simulink model "quadrotor"  (R2019a)
settings: Solver=ode4  StartTime=0.0  StopTime=inf  FixedStep=simparam_delta_t  RelTol=1e-3
model workspace (MAT data in the model file):
  simparam_I = Simulink.Parameter
  simparam_I.Value = [1  0  0; 0  1  0; 0  0  1]
  simparam_I.DataType = 'auto'
  simparam_I.Dimensions = [3 3]
  simparam_delta_t = Simulink.Parameter
  simparam_delta_t.Value = 0.01
  simparam_delta_t.DataType = 'auto'
  simparam_delta_t.Dimensions = [1 1]
  simparam_g = Simulink.Parameter
  simparam_g.Value = 9.81
  simparam_g.DataType = 'auto'
  simparam_g.Dimensions = [1 1]
  simparam_init_euler = Simulink.Parameter
  simparam_init_euler.Value = [0 0 0]
  simparam_init_euler.DataType = 'auto'
  simparam_init_euler.Dimensions = [1 3]
  simparam_init_omega = Simulink.Parameter
  simparam_init_omega.Value = [0 0 0]
  simparam_init_omega.DataType = 'auto'
  simparam_init_omega.Dimensions = [1 3]
  simparam_init_pos = Simulink.Parameter
  simparam_init_pos.Value = [0 0 0]
  simparam_init_pos.DataType = 'auto'
  simparam_init_pos.Dimensions = [1 3]
  simparam_init_rpm = Simulink.Parameter
  simparam_init_rpm.Value = [0 0 0 0]
  simparam_init_rpm.DataType = 'auto'
  simparam_init_rpm.Dimensions = [1 4]
  simparam_init_vel = Simulink.Parameter
  simparam_init_vel.Value = [0 0 0]
  simparam_init_vel.DataType = 'auto'
  simparam_init_vel.Dimensions = [1 3]
  simparam_kq = Simulink.Parameter
  simparam_kq.Value = 0.2
  simparam_kq.DataType = 'auto'
  simparam_kq.Dimensions = [1 1]
  simparam_kt = Simulink.Parameter
  simparam_kt.Value = 0.2
  simparam_kt.DataType = 'auto'
  simparam_kt.Dimensions = [1 1]
  simparam_m = Simulink.Parameter
  simparam_m.Value = 0.5
  simparam_m.DataType = 'auto'
  simparam_m.Dimensions = [1 1]
  simparam_r = Simulink.Parameter
  simparam_r.Value = 0.25
  simparam_r.DataType = 'auto'
  simparam_r.Dimensions = [1 1]
  simparam_tau = Simulink.Parameter
  simparam_tau.Value = 0.05
  simparam_tau.DataType = 'auto'
  simparam_tau.Dimensions = [1 1]
libraries: shared6dof x1, sharedtransform x1
settings Model: OrderedModelArguments=off  Creator=e84872  LastModifiedBy=Alex
settings DataIOCC: ReturnWorkspaceOutputs=off
settings OptimizationCC: DefaultParameterBehavior=Inlined  GainParamInheritBuiltInType=on  UseFloatMulNetSlope=on  InlineInvariantSignals=on  EnhancedBackFolding=on  PassReuseOutputArgsThreshold=0  EfficientFloat2IntCast=on  OptimizeBlockOrder=speed  DifferentSizesBufferReuse=on  OptimizationCustomize=off
settings DebuggingCC: ParameterTunabilityLossMsg=error  ArithmeticOperatorsInVariantConditions=warning
settings SFSimCC: MATLABDynamicMemAlloc=off
settings RTWCC: GenCodeOnly=on  Description=Generic Real-Time Target  GenerateReport=on  Toolchain=MinGW64 | gmake (64-bit Windows)  BuildConfiguration=Faster Runs  LaunchReport=on
settings CodeAppCC: ForceParamTrailComments=on  OperatorAnnotations=on
settings GRTTargetCC: MatFileLogging=off  SupportNonFinite=off

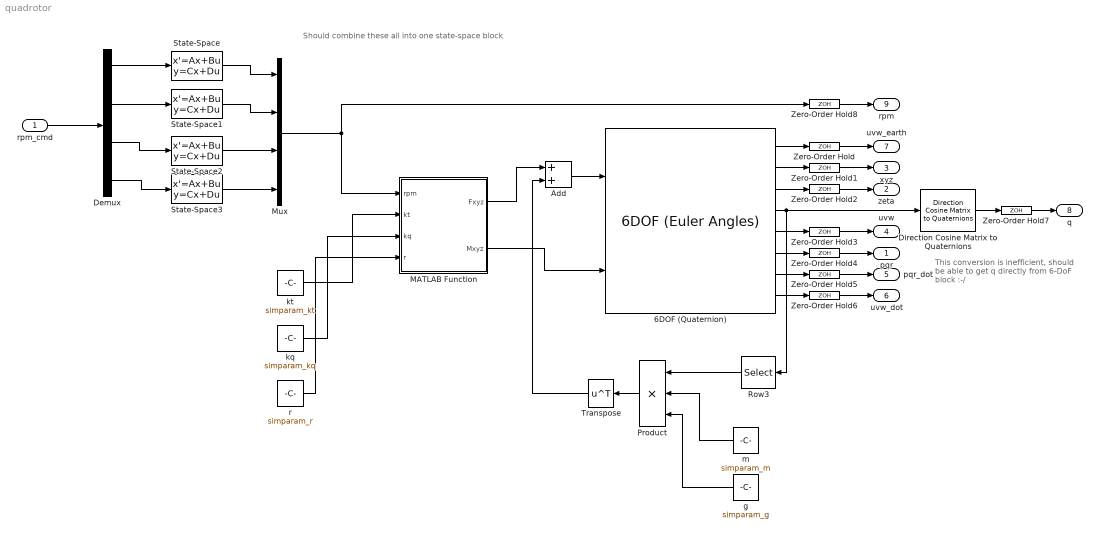
== system quadrotor ==
  note: This conversion is inefficient,
      | should be able to get q directly from
      | 6-DoF block :-/
  note: Should combine these all into one state-space block
  rpm_cmd : Inport  PortDimensions=[4 1]
  6DOF (Quaternion) : shared6dof/6DOF (Euler Angles)  units=Metric (MKS)  mtype=Fixed  rep=Quaternion  xme_0=simparam_init_pos  Vm_0=simparam_init_vel  eul_0=simparam_init_euler  pm_0=simparam_init_omega  mass_0=simparam_m  mass_e=0.5  mass_f=2.0  inertia=simparam_I  inertia_e=eye(3)  inertia_f=2*eye(3)  k_quat=1  vre_flag=on  abi_flag=off  aMode=0  xme_statename=''  Vm_statename=''  eul_statename=''  quat_statename=''  pm_statename=''  mass_statename=''
      settings: SourceProductBaseCode=AE
  Add : Sum
  Demux : Demux
  Direction Cosine Matrix to Quaternions : sharedtransform/Direction Cosine Matrix  to Quaternions  aMode=0  action=None  tolerance=eps(2)
      settings: SourceProductName=Aerospace Blockset  SourceProductBaseCode=AE
  MATLAB Function : MATLAB Function  TreatAsAtomicUnit=on
  Mux : Mux
  Product : Product  Inputs=3
  Row3 : Selector  NumberOfDimensions=2  InputPortWidth=3  IndexOptions=Index vector (dialog),Select all  Indices=3,1  OutputSizes=1,1
  State-Space : StateSpace  A=-1/simparam_tau  C=1/simparam_tau  D=0  InitialCondition=simparam_init_rpm(1)
  State-Space1 : StateSpace  A=-1/simparam_tau  C=1/simparam_tau  D=0  InitialCondition=simparam_init_rpm(2)
  State-Space2 : StateSpace  A=-1/simparam_tau  C=1/simparam_tau  D=0  InitialCondition=simparam_init_rpm(3)
  State-Space3 : StateSpace  A=-1/simparam_tau  C=1/simparam_tau  D=0  InitialCondition=simparam_init_rpm(4)
  Transpose : Math  Operator=transpose  SaturateOnIntegerOverflow=on
  Zero-Order Hold{,1..8} (9 alike) : ZeroOrderHold  SampleTime=-1
  g : Constant  Value=simparam_g
  kq : Constant  Value=simparam_kq
  kt : Constant  Value=simparam_kt
  m : Constant  Value=simparam_m
  r : Constant  Value=simparam_r
  pqr : Outport
  zeta : Outport  Port=2
  xyz : Outport  Port=3
  uvw : Outport  Port=4
  pqr_dot : Outport  Port=5
  uvw_dot : Outport  Port=6
  uvw_earth : Outport  Port=7
  q : Outport  Port=8
  rpm : Outport  Port=9
  wires:
  MATLAB Function/2(Mxyz) -> 6DOF (Quaternion)/2
  6DOF (Quaternion)/6 -> Zero-Order Hold4/1
  6DOF (Quaternion)/3 -> Zero-Order Hold2/1
  6DOF (Quaternion)/2 -> Zero-Order Hold1/1
  Add/1 -> 6DOF (Quaternion)/1
  MATLAB Function/1(Fxyz) -> Add/1
  6DOF (Quaternion)/4 -> Direction Cosine Matrix to Quaternions/1, Row3/1
  Row3/1 -> Product/1
  m/1 -> Product/2
  g/1 -> Product/3
  kt/1 -> MATLAB Function/2(kt)
  kq/1 -> MATLAB Function/3(kq)
  r/1 -> MATLAB Function/4(r)
  Product/1 -> Transpose/1
  Transpose/1 -> Add/2
  rpm_cmd/1 -> Demux/1
  Demux/1 -> State-Space/1
  Demux/2 -> State-Space1/1
  Demux/3 -> State-Space2/1
  Demux/4 -> State-Space3/1
  State-Space/1 -> Mux/1
  State-Space1/1 -> Mux/2
  State-Space2/1 -> Mux/3
  Mux/1 -> MATLAB Function/1(rpm), Zero-Order Hold8/1
  6DOF (Quaternion)/5 -> Zero-Order Hold3/1
  6DOF (Quaternion)/7 -> Zero-Order Hold5/1
  6DOF (Quaternion)/8 -> Zero-Order Hold6/1
  6DOF (Quaternion)/1 -> Zero-Order Hold/1
  Zero-Order Hold/1 -> uvw_earth/1
  Zero-Order Hold1/1 -> xyz/1
  Zero-Order Hold2/1 -> zeta/1
  Zero-Order Hold3/1 -> uvw/1
  Zero-Order Hold4/1 -> pqr/1
  Zero-Order Hold5/1 -> pqr_dot/1
  Zero-Order Hold6/1 -> uvw_dot/1
  Direction Cosine Matrix to Quaternions/1 -> Zero-Order Hold7/1
  Zero-Order Hold7/1 -> q/1
  Zero-Order Hold8/1 -> rpm/1
  State-Space3/1 -> Mux/4

== matlab function quadrotor/MATLAB Function ==
  data: rpm input; Fxyz output; Mxyz output; kt input; kq input; r input
function [Fxyz, Mxyz] = fcn(rpm, kt, kq, r)

% Quadrotor has X-configuration, motors numbered clockwise from front left

omega_squared = (rpm/60*2*pi).^2;

T = kt*omega_squared;
Q = kq*omega_squared;

Fxyz = [0; 0; -sum(T)];
Mxyz = [(T(1) - T(2) - T(3) + T(4))*r; (T(1) + T(2) - T(3) - T(4))*r; -Q(1) + Q(2) - Q(3) + Q(4)];


end
